simulink model "VSG1_RL"  (R2022a)
settings: Solver=FixedStepAuto  StartTime=0.5  StopTime=1  FixedStep=1e-6  RelTol=1e-3
values from neighbouring files (symbols this model uses):
  A5 = [0.002 0.002 0.002 0.002 0.002 0.002 0.002 0.002 0.002 0.002 0.002 0.002 ... (500 elements, 1x500)]    [Am.mat]
  Dmax = 50    [VSG_RL.m]
  Dmin = 20    [VSG_RL.m]
undefined symbols (not defined in the file or in its folder): sigbuilder_block
libraries: slpidlib x4, spsThreePhaseVIMeasurementLib x4, simulink x3, spsabctodq0Lib x3, spsThreePhaseSeriesRLCBranchLib x3, spsGroundLib x2, spsDCVoltageSourceLib x1, spsUniversalBridgeLib x1, powerlib_extras x1, rllib x1, spsThreePhaseSeriesRLCLoadLib x1, spsThreePhaseProgrammableVoltageSourceLib x1
settings Model: SimulationMode=accelerator  Creator=TC  LastModifiedBy=卢闯
settings SolverCC: ZeroCrossAlgorithm=Adaptive  AlgebraicLoopSolver=TrustRegion
settings DataIOCC: InitialState=xFinal  LoadInitialState=on  SaveOperatingPoint=on  SaveOutput=off  SignalLogging=off  DSMLogging=off  SaveTime=off
settings DebuggingCC: IgnoredZcDiagnostic=none  UnconnectedInputMsg=warning  UnconnectedOutputMsg=warning  UnconnectedLineMsg=warning  ArithmeticOperatorsInVariantConditions=warning
settings SFSimCC: CustomCodeUndefinedFunction=UseInterfaceOnly  SimTargetLang=C++  GPUAcceleration=on  SimDLTargetLibrary=cudnn
settings SimscapeCC: SimscapeLogLimitData=off

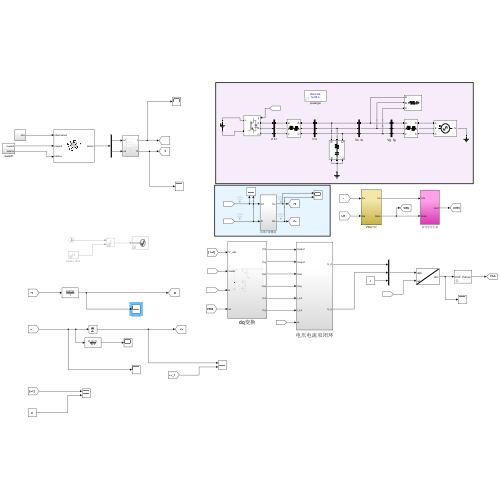
[thumbnail: Simulink's stored preview of the top-level diagram]
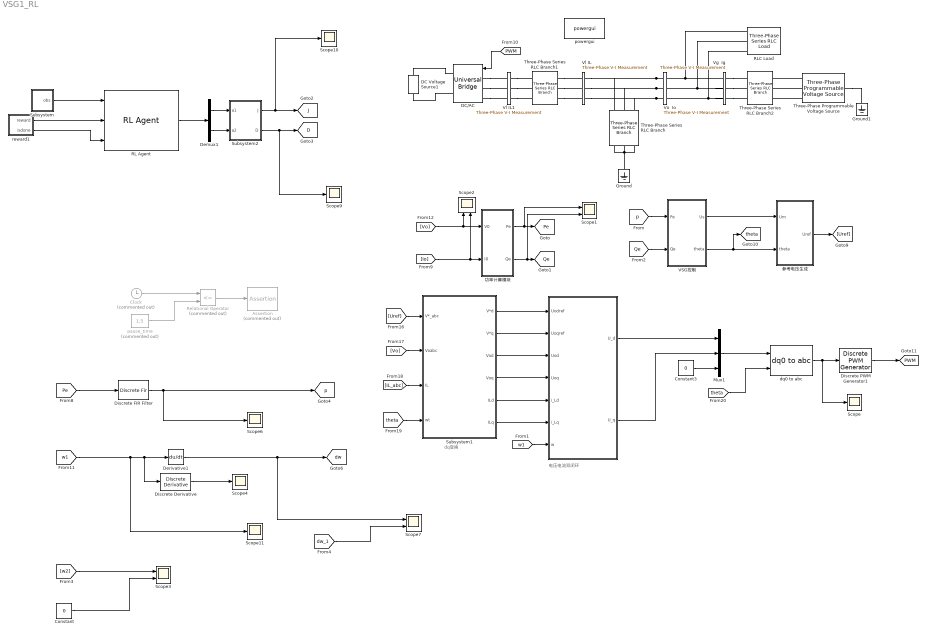
== system VSG1_RL ==
  note: 电压电流双闭环
  note: dq变换
  " " : Subsystem
  Assertion : Assertion  Commented=on  AssertionFailFcn=set_param(bdroot, 'SimulationCommand', 'pause')  StopWhenAssertionFail=off
  Clock : Clock  Commented=on
  Constant : Constant  Value=0
  Constant3 : Constant  Value=0
  DC Voltage Source1 : spsDCVoltageSourceLib/DC Voltage Source  Amplitude=750  Measurements=None
  DC/AC : spsUniversalBridgeLib/Universal Bridge  Arms=3  SnubberResistance=1e5  SnubberCapacitance=inf  Device=IGBT / Diodes  Ron=1e-3  Lon=0  ForwardVoltages="[  0  0  ]"  ForwardVoltage=0  GTOparameters=[ 10e-6 , 20e-6 ]  IGBTparameters=[ 1e-6 , 2e-6 ]  Measurements=None  Measurements_2=None  converterType=Rectifier
  Demux1 : Demux  Outputs=2
  Derivative1 : Derivative
  Discrete PWM Generator1 : powerlib_extras/Discrete  Control Blocks/Discrete PWM Generator  GeneratorMode="3-arm  bridge (6 pulses)"  Fc=10000  Ts=5e-6  Internal=off  mIndex=0.4  Freq=60  Phase=0
      settings: SourceProductBaseCode=PS
  Discrete Derivative : simulink/Discrete/Discrete Derivative  gainval=1.0  ICPrevScaledInput=0.0  OutMin=[]  OutMax=[]  OutDataType=fixdt(1, 16)  OutScaling=2^-10  DoSatur=off
  Discrete FIR Filter : DiscreteFir  Coefficients=A5
  Ground : spsGroundLib/Ground  LConnTagsString=a
  Ground1 : spsGroundLib/Ground  LConnTagsString=a
  Mux1 : Mux  Inputs=3
  RL Agent : rllib/RL Agent  Agent=agent  ExternalActionAsInput=off  ProvideLastAction=off  ProvideCumRwd=off  TreatAsDirectFeedthrough=on  UseStrictObservationDataTypes=off
  RLC Load : spsThreePhaseSeriesRLCLoadLib/Three-Phase Series RLC Load  LConnTagsString=A|B|C  Configuration=Y (grounded)  NominalVoltage=380  Vabc=[1e3 1e3 1e3]  Vabcp=[1e3 1e3 1e3]  NominalFrequency=50  UnbalancedPower=off  ActivePower=10e3  InductivePower=0  CapacitivePower=0  Pabc=[10e3 9e3 11e3]  QLabc=[100 90 110]  QCabc=[100 90 110]  Pabcp=[10e3 9e3 11e3]  QLabcp=[100 90 110]  QCabcp=[100 90 110]  Measurements=Branch voltages and currents  LoadType=constant Z
  Relational Operator : RelationalOperator  Commented=on  Operator=<=  OutDataTypeStr=boolean  RndMeth=Simplest  InputSameDT=off
  Scope{,4,6,9..11} (6 alike) : Scope
  Scope{1..3,7} (4 alike) : Scope  NumInputPorts=2
  Subsystem : Subsystem
  Subsystem1 : Subsystem
  Subsystem2 : Subsystem
  Three-Phase Programmable Voltage Source : spsThreePhaseProgrammableVoltageSourceLib/Three-Phase Programmable Voltage Source  PositiveSequence="[380  0 50]"  VariationEntity=None  VariationType=Table of time-amplitude pairs  VariationTypeAlt=Step  VariationStep=0.5  VariationRate=10  VariationMagnitude=0.3  VariationFrequency=2  VariationTiming=[1 2]  VariationPhaseA=off  Amplitudes=[1 0.8 1.2 1.0]  TimeValues=[0 0.1 0.15 0.2]  HarmonicGeneration=off  HarmonicA=[3 0.2 -25 0]  HarmonicB=[2 0.15 35 2]  Timing="[0.05  3]"  BusType=swing  Pref=0  Qref=0  Qmin=-inf  Qmax=inf
      link override Model/Signal generator/Stair Generator: t=[0.5,1,3,3.5]
  Three-Phase Series RLC Branch : spsThreePhaseSeriesRLCBranchLib/Three-Phase Series RLC Branch  LConnTagsString=A|B|C  RConnTagsString=A|B|C  BranchType=RC  Resistance=1  Inductance=1e-3  Capacitance=20e-6  Measurements=Branch voltages
  Three-Phase Series RLC Branch1 : spsThreePhaseSeriesRLCBranchLib/Three-Phase Series RLC Branch  LConnTagsString=A|B|C  RConnTagsString=A|B|C  BranchType=RL  Resistance=0.1  Inductance=3.2e-3  Capacitance=4.5e-3  Measurements=Branch voltages
  Three-Phase Series RLC Branch2 : spsThreePhaseSeriesRLCBranchLib/Three-Phase Series RLC Branch  LConnTagsString=A|B|C  RConnTagsString=A|B|C  BranchType=RL  Resistance=0.1  Inductance=3.0e-3  Capacitance=4.5e-3  Measurements=Branch voltages
  VSG控制 : Subsystem
  Vg  Ig : spsThreePhaseVIMeasurementLib/Three-Phase V-I Measurement  VoltageMeasurement=phase-to-ground  SetLabelV=on  LabelV=VGG  Vpu=off  VpuLL=off  CurrentMeasurement=yes  SetLabelI=on  LabelI=IGG  Ipu=off  Pbase=Pnom  Vbase=380  OutputType=Complex  PhasorSimulation=off  PSBequivalent=0
  Vl IL : spsThreePhaseVIMeasurementLib/Three-Phase V-I Measurement  VoltageMeasurement=phase-to-ground  SetLabelV=on  LabelV=VL_abc  Vpu=off  VpuLL=off  CurrentMeasurement=yes  SetLabelI=on  LabelI=IL_abc  Ipu=off  Pbase=100e6  Vbase=500e3  OutputType=Complex  PhasorSimulation=off  PSBequivalent=0
  Vl IL1 : spsThreePhaseVIMeasurementLib/Three-Phase V-I Measurement  VoltageMeasurement=phase-to-ground  SetLabelV=on  LabelV=VL  Vpu=off  VpuLL=off  CurrentMeasurement=yes  SetLabelI=on  LabelI=IL  Ipu=off  Pbase=100e6  Vbase=500e3  OutputType=Complex  PhasorSimulation=off  PSBequivalent=0
  Vo  Io : spsThreePhaseVIMeasurementLib/Three-Phase V-I Measurement  VoltageMeasurement=phase-to-ground  SetLabelV=on  LabelV=Vo  Vpu=off  VpuLL=off  CurrentMeasurement=yes  SetLabelI=on  LabelI=Io  Ipu=off  Pbase=Pnom  Vbase=380  OutputType=Complex  PhasorSimulation=off  PSBequivalent=0
  dq0 to abc : spsdq0toabcLib/dq0 to abc  Alignment=90 degrees behind phase A axis
  pause_time : Constant  Commented=on  Value=1.5
  powergui : spspowerguiLib/powergui  Priority=1  SimulationMode=Discrete  SampleTime=1e-6  frequency=60  Iterations=50  frequencyindice=0  Pbase=100e6  ErrMax=1e-4  UnitsV=kV  UnitsW=MW  buscounter=0  FunctionMessages=off  echomessages=off  EnableUseOfTLC=off  CurrentSourceSwitches=off  DisableSnubberDevices=off  DisableRonSwitches=off  DisableVfSwitches=off  DisplayEquations=off  AutomaticDiscreteSolvers=off  SolverType=Tustin/Backward Euler (TBE)  Interpol=off  ExternalGateDelay=off  methode=off  Ts=100  x0status=blocks  SPID=on  SwTol=0  HookPort=off  NonlinearTolerance=1e-4  nMaxIteration=100  ContinueOnMaxIteration=off  RestoreLinks=warning  ResistiveCurrentMeasurement=off  Frange=[0:2:500]  Ylog=off  Xlog=on  ShowGrid=off  save=off  variable=ZData  structure=0  ZoomFFT=off  StartTime=0.0  cycles=1  DisplayStyle=1  fundamental=60  FreqAxis=off  MaxFrequency=1000  frequencyindicesteady=1  RmsSteady=1  display=off
  reward1 : Subsystem
  功率计算模块 : Subsystem
  参考电压生成 : Subsystem
  tag scope: D=global, J=global, PWM=global, Pe=global, Qe=global, dw=global, p=global, theta=global
  wires:
  [PWM] -> DC/AC/1
  Mux1/1 -> dq0 to abc/1
  dq0 to abc/1 -> Scope/1, Discrete PWM Generator1/1
  " "/2(U_q) -> Mux1/2
  Discrete PWM Generator1/1 -> [PWM]
  参考电压生成/1(Uref) -> [Uref]
  [w1] -> " "/7(w)
  [IL_abc] -> Subsystem1/3(IL)
  [theta] -> Subsystem1/4(wt)
  Subsystem1/4(Voq) -> " "/4(Uoq)
  [Uref] -> Subsystem1/1(V*_abc)
  [theta] -> dq0 to abc/2
  [Io] -> 功率计算模块/2(I0), Scope2/2
  Constant3/1 -> Mux1/3
  " "/1(U_d) -> Mux1/1
  Subsystem1/1(V*d) -> " "/1(Uodref)
  [Vo] -> Subsystem1/2(Voabc)
  Subsystem1/2(V*q) -> " "/2(Uoqref)
  VSG控制/2(theta) -> 参考电压生成/2(theta), [theta]
  Subsystem1/5(ILd) -> " "/5(i_Ld)
  Subsystem1/3(Vod) -> " "/3(Uod)
  Subsystem1/6(ILq) -> " "/6(i_Lq)
  [Vo] -> 功率计算模块/1(V0), Scope2/1
  VSG控制/1(Us) -> 参考电压生成/1(Um)
  功率计算模块/1(Pe) -> Scope1/1, [Pe]
  功率计算模块/2(Qe) -> Scope1/2, [Qe]
  [p] -> VSG控制/1(Pe)
  [Qe] -> VSG控制/2(Qe)
  Clock/1 -> Relational Operator/1
  pause_time/1 -> Relational Operator/2
  Relational Operator/1 -> Assertion/1
  [w1] -> Discrete Derivative/1, Derivative1/1, Scope11/1
  [Pe] -> Discrete FIR Filter/1
  Discrete FIR Filter/1 -> [p], Scope6/1
  Subsystem2/2(D) -> Scope9/1, [D]
  Subsystem2/1(J) -> Scope10/1, [J]
  Demux1/1 -> Subsystem2/1(a1)
  Demux1/2 -> Subsystem2/2(a2)
  Subsystem/1(obs) -> RL Agent/1
  RL Agent/1 -> Demux1/1
  Derivative1/1 -> [dw], Scope7/1
  [w2] -> Scope3/1
  Constant/1 -> Scope3/2
  reward1/1(reward) -> RL Agent/2
  Discrete Derivative/1 -> Scope4/1
  [dw_1] -> Scope7/2
  reward1/2(isdone) -> RL Agent/3
  connections:
  Ground/LConn1 -- Three-Phase Series RLC Branch/RConn2 -- Three-Phase Series RLC Branch/RConn3 -- Three-Phase Series RLC Branch/RConn1
  Vo  Io/LConn2 -- Vl IL/RConn2 -- Three-Phase Series RLC Branch/LConn2
  Vo  Io/LConn3 -- Vl IL/RConn3 -- Three-Phase Series RLC Branch/LConn3
  Vo  Io/LConn1 -- Vl IL/RConn1 -- Three-Phase Series RLC Branch/LConn1
  Three-Phase Programmable Voltage Source/RConn3 -- Three-Phase Series RLC Branch2/LConn3
  Vg  Ig/LConn3 -- Vo  Io/RConn3 -- RLC Load/LConn3
  Three-Phase Programmable Voltage Source/RConn2 -- Three-Phase Series RLC Branch2/LConn2
  Three-Phase Series RLC Branch1/LConn2 -- Vl IL/LConn2
  Vg  Ig/LConn1 -- RLC Load/LConn1 -- Vo  Io/RConn1
  Three-Phase Programmable Voltage Source/RConn1 -- Three-Phase Series RLC Branch2/LConn1
  Three-Phase Programmable Voltage Source/LConn1 -- Ground1/LConn1
  Three-Phase Series RLC Branch1/LConn1 -- Vl IL/LConn1
  Vg  Ig/LConn2 -- RLC Load/LConn2 -- Vo  Io/RConn2
  Three-Phase Series RLC Branch1/LConn3 -- Vl IL/LConn3
  Vg  Ig/RConn1 -- Three-Phase Series RLC Branch2/RConn1
  Vg  Ig/RConn2 -- Three-Phase Series RLC Branch2/RConn2
  Vg  Ig/RConn3 -- Three-Phase Series RLC Branch2/RConn3
  DC Voltage Source1/RConn1 -- DC/AC/RConn1
  DC Voltage Source1/LConn1 -- DC/AC/RConn2
  DC/AC/LConn1 -- Vl IL1/LConn1
  Vl IL1/RConn1 -- Three-Phase Series RLC Branch1/RConn1
  DC/AC/LConn2 -- Vl IL1/LConn2
  Vl IL1/RConn2 -- Three-Phase Series RLC Branch1/RConn2
  DC/AC/LConn3 -- Vl IL1/LConn3
  Vl IL1/RConn3 -- Three-Phase Series RLC Branch1/RConn3

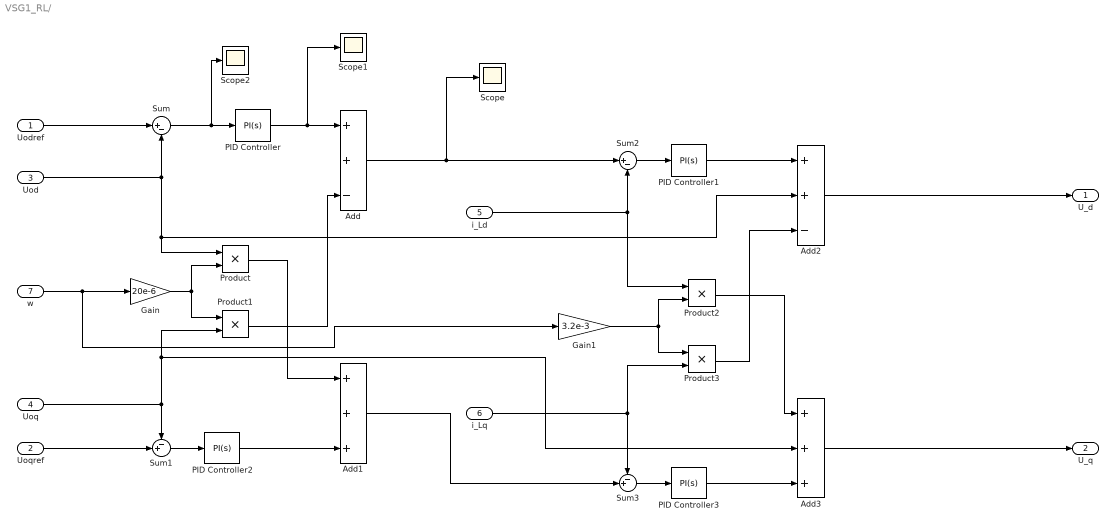
== system VSG1_RL/  ==
  Uodref : Inport
  Uoqref : Inport  Port=2
  Uod : Inport  Port=3
  Uoq : Inport  Port=4
  i_Ld : Inport  Port=5
  i_Lq : Inport  Port=6
  w : Inport  Port=7
  Add : Sum  Inputs=++-
  Add1 : Sum  Inputs=+++
  Add2 : Sum  Inputs=++-
  Add3 : Sum  Inputs=+++
  Gain : Gain  Gain=20e-6
  Gain1 : Gain  Gain=3.2e-3
  PID Controller : slpidlib/PID Controller  Controller=PI  Form=Parallel  TimeDomain=Continuous-time  UseExternalTs=off  SampleTime=1  IntegratorMethod=Forward Euler  FilterMethod=Forward Euler  ControllerParametersSource=internal  P=5  I=250  UseKiTs=off  D=0  N=100  UseFilter=on  TunerSelectOption=Transfer Function Based (PID Tuner App)  InitialConditionSource=internal  InitialConditionForIntegrator=0  InitialConditionForFilter=0  DifferentiatorICPrevScaledInput=0  ExternalReset=none  TrackingMode=off  Kt=1  LimitOutput=off  SatLimitsSource=internal  UpperSaturationLimit=inf  LowerSaturationLimit=-inf  LinearizeAsGain=off  AntiWindupMode=none  Kb=1  POutMin=[]  POutMax=[]  IOutMin=[]  IOutMax=[]  DOutMin=[]  DOutMax=[]  NOutMin=[]  NOutMax=[]  SumOutMin=[]  SumOutMax=[]  SaturationOutMin=[]  SaturationOutMax=[]  PParamMin=[]  PParamMax=[]  IParamMin=[]  IParamMax=[]  DParamMin=[]  DParamMax=[]  NParamMin=[]  NParamMax=[]  KbParamMin=[]  KbParamMax=[]  KtParamMin=[]  KtParamMax=[]  KbOutMin=[]  KbOutMax=[]  KtOutMin=[]  KtOutMax=[]  IntegratorOutMin=[]  IntegratorOutMax=[]  FilterOutMin=[]  FilterOutMax=[]  SumI1OutMin=[]  SumI1OutMax=[]  SumI2OutMin=[]  SumI2OutMax=[]  SumI3OutMin=[]  SumI3OutMax=[]  SumI4OutMin=[]  SumI4OutMax=[]  SumDOutMin=[]  SumDOutMax=[]  DifferentiatorOutMin=[]  DifferentiatorOutMax=[]  FilterDiffOutCoefMin=[]  FilterDiffOutCoefMax=[]  ReciprocalOutMin=[]  ReciprocalOutMax=[]  SumDenOutMin=[]  SumDenOutMax=[]  SumNumOutMin=[]  SumNumOutMax=[]  DivideOutMin=[]  DivideOutMax=[]  UdiffTsProdOutMin=[]  UdiffTsProdOutMax=[]  NTsProdOutMin=[]  NTsProdOutMax=[]  UintegralTsProdOutMin=[]  UintegralTsProdOutMax=[]  UngainTsProdOutMin=[]  UngainTsProdOutMax=[]  ClampingZeroOutDataTypeStr=Inherit: Inherit via back propagation  ClampingZeroOutMin=[]  ClampingZeroOutMax=[]  FilterDenConstantOutDataTypeStr=Inherit: Inherit via back propagation  FilterDenConstantOutMin=[]  FilterDenConstantOutMax=[]  PCopyOutDataTypeStr=Inherit: Inherit via back propagation  PCopyOutMin=[]  PCopyOutMax=[]  NCopyOutDataTypeStr=Inherit: Inherit via back propagation  NCopyOutMin=[]  NCopyOutMax=[]  IntegratorContinuousStateAttributes=''  IntegratorStateMustResolveToSignalObject=off  IntegratorRTWStateStorageClass=Auto  FilterContinuousStateAttributes=''  FilterStateMustResolveToSignalObject=off  FilterRTWStateStorageClass=Auto  ParallelPVariant=InternalParameters  IdealPVariant=Disabled  IVariant=InternalParameters  DVariant=Disabled  IntegratorVariant=Continuous  SatVariant=Disabled  AWVariant=Passthrough  PCopyVariant=Disabled  TRVariant=Disabled  FdbkBlocksVariant=Forward  IdealPFdbkVariant=Disabled  SatFdbkVariant=Disabled  DerivativeFilterVariant=Disabled  NVariant=Disabled  NCopyVariant=Disabled_SignalSpec  FilterICVariant=Disabled  IntegratorICVariant=InternalICs  ExternalResetVariant=Disabled  TRSumVariant=Passthrough  SumFdbkVariant=Disabled  SumVariant=Sum_PI  TsampFilterVariant=InternalTs  TsampNgainVariant=Passthrough  TsampIntegralVariant=Passthrough  ExternalSaturationOutDataTypeStr=Inherit: Same as second input  aMode=0
  PID Controller1 : slpidlib/PID Controller  Controller=PI  Form=Parallel  TimeDomain=Continuous-time  UseExternalTs=off  SampleTime=1  IntegratorMethod=Forward Euler  FilterMethod=Forward Euler  ControllerParametersSource=internal  P=20  I=200  UseKiTs=off  D=0  N=100  UseFilter=on  TunerSelectOption=Transfer Function Based (PID Tuner App)  InitialConditionSource=internal  InitialConditionForIntegrator=0  InitialConditionForFilter=0  DifferentiatorICPrevScaledInput=0  ExternalReset=none  TrackingMode=off  Kt=1  LimitOutput=off  SatLimitsSource=internal  UpperSaturationLimit=inf  LowerSaturationLimit=-inf  LinearizeAsGain=off  AntiWindupMode=none  Kb=1  POutMin=[]  POutMax=[]  IOutMin=[]  IOutMax=[]  DOutMin=[]  DOutMax=[]  NOutMin=[]  NOutMax=[]  SumOutMin=[]  SumOutMax=[]  SaturationOutMin=[]  SaturationOutMax=[]  PParamMin=[]  PParamMax=[]  IParamMin=[]  IParamMax=[]  DParamMin=[]  DParamMax=[]  NParamMin=[]  NParamMax=[]  KbParamMin=[]  KbParamMax=[]  KtParamMin=[]  KtParamMax=[]  KbOutMin=[]  KbOutMax=[]  KtOutMin=[]  KtOutMax=[]  IntegratorOutMin=[]  IntegratorOutMax=[]  FilterOutMin=[]  FilterOutMax=[]  SumI1OutMin=[]  SumI1OutMax=[]  SumI2OutMin=[]  SumI2OutMax=[]  SumI3OutMin=[]  SumI3OutMax=[]  SumI4OutMin=[]  SumI4OutMax=[]  SumDOutMin=[]  SumDOutMax=[]  DifferentiatorOutMin=[]  DifferentiatorOutMax=[]  FilterDiffOutCoefMin=[]  FilterDiffOutCoefMax=[]  ReciprocalOutMin=[]  ReciprocalOutMax=[]  SumDenOutMin=[]  SumDenOutMax=[]  SumNumOutMin=[]  SumNumOutMax=[]  DivideOutMin=[]  DivideOutMax=[]  UdiffTsProdOutMin=[]  UdiffTsProdOutMax=[]  NTsProdOutMin=[]  NTsProdOutMax=[]  UintegralTsProdOutMin=[]  UintegralTsProdOutMax=[]  UngainTsProdOutMin=[]  UngainTsProdOutMax=[]  ClampingZeroOutDataTypeStr=Inherit: Inherit via back propagation  ClampingZeroOutMin=[]  ClampingZeroOutMax=[]  FilterDenConstantOutDataTypeStr=Inherit: Inherit via back propagation  FilterDenConstantOutMin=[]  FilterDenConstantOutMax=[]  PCopyOutDataTypeStr=Inherit: Inherit via back propagation  PCopyOutMin=[]  PCopyOutMax=[]  NCopyOutDataTypeStr=Inherit: Inherit via back propagation  NCopyOutMin=[]  NCopyOutMax=[]  IntegratorContinuousStateAttributes=''  IntegratorStateMustResolveToSignalObject=off  IntegratorRTWStateStorageClass=Auto  FilterContinuousStateAttributes=''  FilterStateMustResolveToSignalObject=off  FilterRTWStateStorageClass=Auto  ParallelPVariant=InternalParameters  IdealPVariant=Disabled  IVariant=InternalParameters  DVariant=Disabled  IntegratorVariant=Continuous  SatVariant=Disabled  AWVariant=Passthrough  PCopyVariant=Disabled  TRVariant=Disabled  FdbkBlocksVariant=Forward  IdealPFdbkVariant=Disabled  SatFdbkVariant=Disabled  DerivativeFilterVariant=Disabled  NVariant=Disabled  NCopyVariant=Disabled_SignalSpec  FilterICVariant=Disabled  IntegratorICVariant=InternalICs  ExternalResetVariant=Disabled  TRSumVariant=Passthrough  SumFdbkVariant=Disabled  SumVariant=Sum_PI  TsampFilterVariant=InternalTs  TsampNgainVariant=Passthrough  TsampIntegralVariant=Passthrough  ExternalSaturationOutDataTypeStr=Inherit: Same as second input  aMode=0
  PID Controller2 : slpidlib/PID Controller  Controller=PI  Form=Parallel  TimeDomain=Continuous-time  UseExternalTs=off  SampleTime=1  IntegratorMethod=Forward Euler  FilterMethod=Forward Euler  ControllerParametersSource=internal  P=5  I=250  UseKiTs=off  D=0  N=100  UseFilter=on  TunerSelectOption=Transfer Function Based (PID Tuner App)  InitialConditionSource=internal  InitialConditionForIntegrator=0  InitialConditionForFilter=0  DifferentiatorICPrevScaledInput=0  ExternalReset=none  TrackingMode=off  Kt=1  LimitOutput=off  SatLimitsSource=internal  UpperSaturationLimit=inf  LowerSaturationLimit=-inf  LinearizeAsGain=off  AntiWindupMode=none  Kb=1  POutMin=[]  POutMax=[]  IOutMin=[]  IOutMax=[]  DOutMin=[]  DOutMax=[]  NOutMin=[]  NOutMax=[]  SumOutMin=[]  SumOutMax=[]  SaturationOutMin=[]  SaturationOutMax=[]  PParamMin=[]  PParamMax=[]  IParamMin=[]  IParamMax=[]  DParamMin=[]  DParamMax=[]  NParamMin=[]  NParamMax=[]  KbParamMin=[]  KbParamMax=[]  KtParamMin=[]  KtParamMax=[]  KbOutMin=[]  KbOutMax=[]  KtOutMin=[]  KtOutMax=[]  IntegratorOutMin=[]  IntegratorOutMax=[]  FilterOutMin=[]  FilterOutMax=[]  SumI1OutMin=[]  SumI1OutMax=[]  SumI2OutMin=[]  SumI2OutMax=[]  SumI3OutMin=[]  SumI3OutMax=[]  SumI4OutMin=[]  SumI4OutMax=[]  SumDOutMin=[]  SumDOutMax=[]  DifferentiatorOutMin=[]  DifferentiatorOutMax=[]  FilterDiffOutCoefMin=[]  FilterDiffOutCoefMax=[]  ReciprocalOutMin=[]  ReciprocalOutMax=[]  SumDenOutMin=[]  SumDenOutMax=[]  SumNumOutMin=[]  SumNumOutMax=[]  DivideOutMin=[]  DivideOutMax=[]  UdiffTsProdOutMin=[]  UdiffTsProdOutMax=[]  NTsProdOutMin=[]  NTsProdOutMax=[]  UintegralTsProdOutMin=[]  UintegralTsProdOutMax=[]  UngainTsProdOutMin=[]  UngainTsProdOutMax=[]  ClampingZeroOutDataTypeStr=Inherit: Inherit via back propagation  ClampingZeroOutMin=[]  ClampingZeroOutMax=[]  FilterDenConstantOutDataTypeStr=Inherit: Inherit via back propagation  FilterDenConstantOutMin=[]  FilterDenConstantOutMax=[]  PCopyOutDataTypeStr=Inherit: Inherit via back propagation  PCopyOutMin=[]  PCopyOutMax=[]  NCopyOutDataTypeStr=Inherit: Inherit via back propagation  NCopyOutMin=[]  NCopyOutMax=[]  IntegratorContinuousStateAttributes=''  IntegratorStateMustResolveToSignalObject=off  IntegratorRTWStateStorageClass=Auto  FilterContinuousStateAttributes=''  FilterStateMustResolveToSignalObject=off  FilterRTWStateStorageClass=Auto  ParallelPVariant=InternalParameters  IdealPVariant=Disabled  IVariant=InternalParameters  DVariant=Disabled  IntegratorVariant=Continuous  SatVariant=Disabled  AWVariant=Passthrough  PCopyVariant=Disabled  TRVariant=Disabled  FdbkBlocksVariant=Forward  IdealPFdbkVariant=Disabled  SatFdbkVariant=Disabled  DerivativeFilterVariant=Disabled  NVariant=Disabled  NCopyVariant=Disabled_SignalSpec  FilterICVariant=Disabled  IntegratorICVariant=InternalICs  ExternalResetVariant=Disabled  TRSumVariant=Passthrough  SumFdbkVariant=Disabled  SumVariant=Sum_PI  TsampFilterVariant=InternalTs  TsampNgainVariant=Passthrough  TsampIntegralVariant=Passthrough  ExternalSaturationOutDataTypeStr=Inherit: Same as second input  aMode=0
  PID Controller3 : slpidlib/PID Controller  Controller=PI  Form=Parallel  TimeDomain=Continuous-time  UseExternalTs=off  SampleTime=1  IntegratorMethod=Forward Euler  FilterMethod=Forward Euler  ControllerParametersSource=internal  P=20  I=200  UseKiTs=off  D=0  N=100  UseFilter=on  TunerSelectOption=Transfer Function Based (PID Tuner App)  InitialConditionSource=internal  InitialConditionForIntegrator=0  InitialConditionForFilter=0  DifferentiatorICPrevScaledInput=0  ExternalReset=none  TrackingMode=off  Kt=1  LimitOutput=off  SatLimitsSource=internal  UpperSaturationLimit=inf  LowerSaturationLimit=-inf  LinearizeAsGain=off  AntiWindupMode=none  Kb=1  POutMin=[]  POutMax=[]  IOutMin=[]  IOutMax=[]  DOutMin=[]  DOutMax=[]  NOutMin=[]  NOutMax=[]  SumOutMin=[]  SumOutMax=[]  SaturationOutMin=[]  SaturationOutMax=[]  PParamMin=[]  PParamMax=[]  IParamMin=[]  IParamMax=[]  DParamMin=[]  DParamMax=[]  NParamMin=[]  NParamMax=[]  KbParamMin=[]  KbParamMax=[]  KtParamMin=[]  KtParamMax=[]  KbOutMin=[]  KbOutMax=[]  KtOutMin=[]  KtOutMax=[]  IntegratorOutMin=[]  IntegratorOutMax=[]  FilterOutMin=[]  FilterOutMax=[]  SumI1OutMin=[]  SumI1OutMax=[]  SumI2OutMin=[]  SumI2OutMax=[]  SumI3OutMin=[]  SumI3OutMax=[]  SumI4OutMin=[]  SumI4OutMax=[]  SumDOutMin=[]  SumDOutMax=[]  DifferentiatorOutMin=[]  DifferentiatorOutMax=[]  FilterDiffOutCoefMin=[]  FilterDiffOutCoefMax=[]  ReciprocalOutMin=[]  ReciprocalOutMax=[]  SumDenOutMin=[]  SumDenOutMax=[]  SumNumOutMin=[]  SumNumOutMax=[]  DivideOutMin=[]  DivideOutMax=[]  UdiffTsProdOutMin=[]  UdiffTsProdOutMax=[]  NTsProdOutMin=[]  NTsProdOutMax=[]  UintegralTsProdOutMin=[]  UintegralTsProdOutMax=[]  UngainTsProdOutMin=[]  UngainTsProdOutMax=[]  ClampingZeroOutDataTypeStr=Inherit: Inherit via back propagation  ClampingZeroOutMin=[]  ClampingZeroOutMax=[]  FilterDenConstantOutDataTypeStr=Inherit: Inherit via back propagation  FilterDenConstantOutMin=[]  FilterDenConstantOutMax=[]  PCopyOutDataTypeStr=Inherit: Inherit via back propagation  PCopyOutMin=[]  PCopyOutMax=[]  NCopyOutDataTypeStr=Inherit: Inherit via back propagation  NCopyOutMin=[]  NCopyOutMax=[]  IntegratorContinuousStateAttributes=''  IntegratorStateMustResolveToSignalObject=off  IntegratorRTWStateStorageClass=Auto  FilterContinuousStateAttributes=''  FilterStateMustResolveToSignalObject=off  FilterRTWStateStorageClass=Auto  ParallelPVariant=InternalParameters  IdealPVariant=Disabled  IVariant=InternalParameters  DVariant=Disabled  IntegratorVariant=Continuous  SatVariant=Disabled  AWVariant=Passthrough  PCopyVariant=Disabled  TRVariant=Disabled  FdbkBlocksVariant=Forward  IdealPFdbkVariant=Disabled  SatFdbkVariant=Disabled  DerivativeFilterVariant=Disabled  NVariant=Disabled  NCopyVariant=Disabled_SignalSpec  FilterICVariant=Disabled  IntegratorICVariant=InternalICs  ExternalResetVariant=Disabled  TRSumVariant=Passthrough  SumFdbkVariant=Disabled  SumVariant=Sum_PI  TsampFilterVariant=InternalTs  TsampNgainVariant=Passthrough  TsampIntegralVariant=Passthrough  ExternalSaturationOutDataTypeStr=Inherit: Same as second input  aMode=0
  Product{,1..3} (4 alike) : Product  RndMeth=Zero
  Scope : Scope
  Scope1 : Scope
  Scope2 : Scope
  Sum : Sum  Inputs=|+-
  Sum1 : Sum  Inputs=-+|
  Sum2 : Sum  Inputs=|+-
  Sum3 : Sum  Inputs=-+|
  U_d : Outport  VectorParamsAs1DForOutWhenUnconnected=off
  U_q : Outport  Port=2  VectorParamsAs1DForOutWhenUnconnected=off
  wires:
  Uod/1 -> Sum/2, Add2/2, Product/1
  Add/1 -> Scope/1, Sum2/1
  i_Lq/1 -> Sum3/1, Product3/2
  i_Ld/1 -> Sum2/2, Product2/1
  Sum2/1 -> PID Controller1/1
  PID Controller1/1 -> Add2/1
  Add1/1 -> Sum3/2
  Product2/1 -> Add3/1
  Product3/1 -> Add2/3
  Gain/1 -> Product1/1, Product/2
  Gain1/1 -> Product3/1, Product2/2
  Uoq/1 -> Sum1/1, Product1/2, Add3/2
  PID Controller3/1 -> Add3/3
  Sum3/1 -> PID Controller3/1
  Product1/1 -> Add/3
  Product/1 -> Add1/1
  PID Controller2/1 -> Add1/3
  Sum1/1 -> PID Controller2/1
  PID Controller/1 -> Scope1/1, Add/1
  w/1 -> Gain1/1, Gain/1
  Uoqref/1 -> Sum1/2
  Uodref/1 -> Sum/1
  Sum/1 -> Scope2/1, PID Controller/1
  Add2/1 -> U_d/1
  Add3/1 -> U_q/1

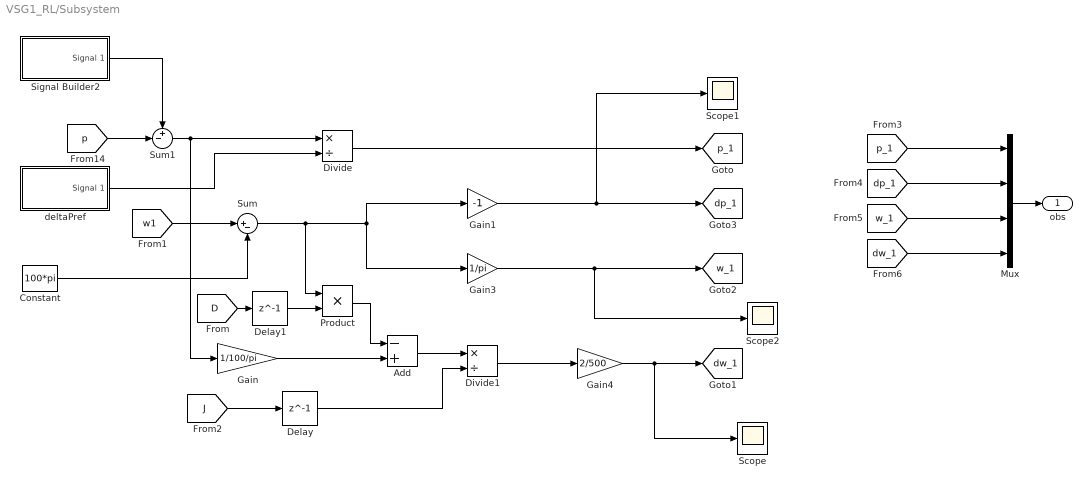
== system VSG1_RL/Subsystem ==
  Add : Sum  Inputs=-+
  Constant : Constant  Value=100*pi
  Delay : Delay  DelayLength=1  InitialCondition=0.02  SampleTime=0.0005
  Delay1 : Delay  DelayLength=1  SampleTime=0.0005
  Divide : Product  Inputs=*/
  Divide1 : Product  Inputs=*/
  Gain : Gain  Gain=1/100/pi
  Gain1 : Gain  Gain=-1
  Gain3 : Gain  Gain=1/pi
  Gain4 : Gain  Gain=2/500
  Mux : Mux
  Product : Product
  Scope : Scope
  Scope1 : Scope
  Scope2 : Scope
  Signal Builder2 : Subsystem  Tag=STV Subsys  LoadFcn=sigbuilder_block('load');  StartFcn=sigbuilder_block('start');  StopFcn=sigbuilder_block('stop');  ClipboardFcn=sigbuilder_block('clipboard');  mask(Sigbuilder block){tuvar=[0:10]}
      mask help: Simulink:masks:SigbuilderBlock_MD
      mask init:
      | if ~strcmp(get_param(bdroot(gcbh),'SimulationStatus'),'stopped') tuvar = sigbuilder_block('maskInit'); end
      settings: CopyFcn=sigbuilder_block('copy');  DeleteFcn=sigbuilder_block('delete');  ModelCloseFcn=sigbuilder_block('modelClose');  PreSaveFcn=sigbuilder_block('preSave');  PauseFcn=sigbuilder_block('pause');  ContinueFcn=sigbuilder_block('continue');  NameChangeFcn=sigbuilder_block('namechange');  OpenFcn=sigbuilder_block('open',[63 119.25 1012.5 505.5 ]);  CloseFcn=sigbuilder_block('close');
      mask Display: plot(0, 0, 100, 100,[2, 2, 32, 32, 2], [68, 8, 8, 68, 68],[32, 2], [38, 38], [32, 19, 2],[53, 60, 44], [32, 17, 17, 2],[16, 16, 31, 31]);txt = getActiveGroup(gcbh);text(2, 100, txt,'verticalAlignment', 'top');
  Sum : Sum  Inputs=|+-
  Sum1 : Sum  Inputs=+-|
  deltaPref : Subsystem  Tag=STV Subsys  LoadFcn=sigbuilder_block('load');  StartFcn=sigbuilder_block('start');  StopFcn=sigbuilder_block('stop');  ClipboardFcn=sigbuilder_block('clipboard');  mask(Sigbuilder block){tuvar=[0:10]}
      mask help: Simulink:masks:SigbuilderBlock_MD
      mask init:
      | if ~strcmp(get_param(bdroot(gcbh),'SimulationStatus'),'stopped') tuvar = sigbuilder_block('maskInit'); end
      settings: CopyFcn=sigbuilder_block('copy');  DeleteFcn=sigbuilder_block('delete');  ModelCloseFcn=sigbuilder_block('modelClose');  PreSaveFcn=sigbuilder_block('preSave');  PauseFcn=sigbuilder_block('pause');  ContinueFcn=sigbuilder_block('continue');  NameChangeFcn=sigbuilder_block('namechange');  OpenFcn=sigbuilder_block('open',[63 119.25 1012.5 505.5 ]);  CloseFcn=sigbuilder_block('close');
      mask Display: plot(0, 0, 100, 100,[2, 2, 32, 32, 2], [68, 8, 8, 68, 68],[32, 2], [38, 38], [32, 19, 2],[53, 60, 44], [32, 17, 17, 2],[16, 16, 31, 31]);txt = getActiveGroup(gcbh);text(2, 100, txt,'verticalAlignment', 'top');
  obs : Outport
  tag scope: dp_1=global, dw_1=global, p_1=global, w_1=global
  wires:
  Signal Builder2/1(Signal 1) -> Sum1/1
  [p] -> Sum1/2
  Mux/1 -> obs/1
  [w1] -> Sum/1
  Sum/1 -> Product/1, Gain1/1, Gain3/1
  Constant/1 -> Sum/2
  Gain3/1 -> Scope2/1, [w_1]
  Sum1/1 -> Gain/1, Divide/1
  deltaPref/1(Signal 1) -> Divide/2
  Divide/1 -> [p_1]
  [D] -> Delay1/1
  Gain/1 -> Add/2
  Product/1 -> Add/1
  Add/1 -> Divide1/1
  [J] -> Delay/1
  Gain1/1 -> Scope1/1, [dp_1]
  Divide1/1 -> Gain4/1
  [p_1] -> Mux/1
  [dp_1] -> Mux/2
  [w_1] -> Mux/3
  [dw_1] -> Mux/4
  Delay/1 -> Divide1/2
  Delay1/1 -> Product/2
  Gain4/1 -> Scope/1, [dw_1]

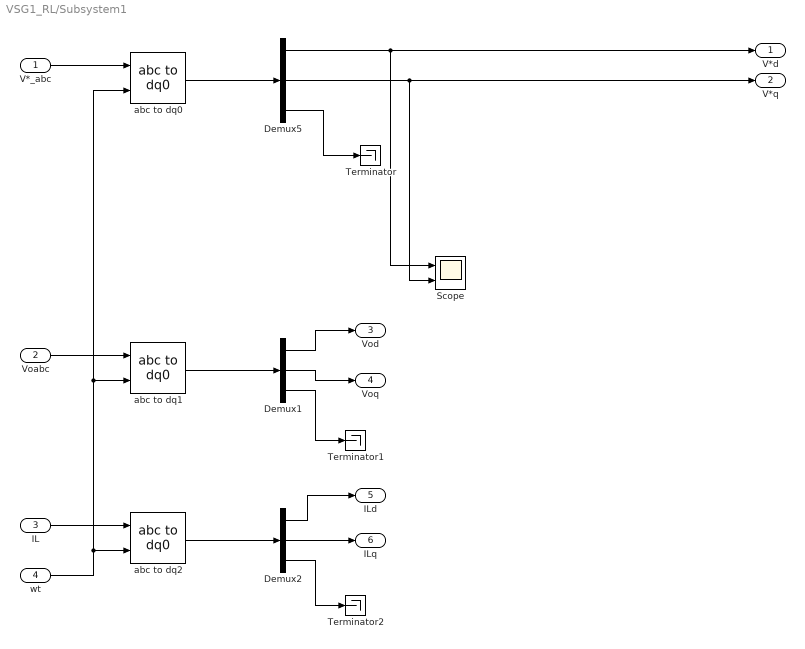
== system VSG1_RL/Subsystem1 ==
  V*_abc : Inport
  Voabc : Inport  Port=2
  IL : Inport  Port=3
  wt : Inport  Port=4
  Demux1 : Demux  Outputs=3
  Demux2 : Demux  Outputs=3
  Demux5 : Demux  Outputs=3
  Scope : Scope  NumInputPorts=2
  Terminator : Terminator
  Terminator1 : Terminator
  Terminator2 : Terminator
  abc to dq0 : spsabctodq0Lib/abc to dq0  Alignment=90 degrees behind phase A axis
  abc to dq1 : spsabctodq0Lib/abc to dq0  Alignment=90 degrees behind phase A axis
  abc to dq2 : spsabctodq0Lib/abc to dq0  Alignment=90 degrees behind phase A axis
  V*d : Outport  VectorParamsAs1DForOutWhenUnconnected=off
  V*q : Outport  Port=2  VectorParamsAs1DForOutWhenUnconnected=off
  Vod : Outport  Port=3  VectorParamsAs1DForOutWhenUnconnected=off
  Voq : Outport  Port=4  VectorParamsAs1DForOutWhenUnconnected=off
  ILd : Outport  Port=5  VectorParamsAs1DForOutWhenUnconnected=off
  ILq : Outport  Port=6  VectorParamsAs1DForOutWhenUnconnected=off
  wires:
  Demux5/2 -> V*q/1, Scope/2
  Demux5/1 -> V*d/1, Scope/1
  IL/1 -> abc to dq2/1
  Demux2/2 -> ILq/1
  Demux1/2 -> Voq/1
  Demux1/1 -> Vod/1
  Demux2/3 -> Terminator2/1
  Demux5/3 -> Terminator/1
  V*_abc/1 -> abc to dq0/1
  wt/1 -> abc to dq0/2, abc to dq1/2, abc to dq2/2
  Voabc/1 -> abc to dq1/1
  abc to dq1/1 -> Demux1/1
  abc to dq2/1 -> Demux2/1
  Demux1/3 -> Terminator1/1
  abc to dq0/1 -> Demux5/1
  Demux2/1 -> ILd/1

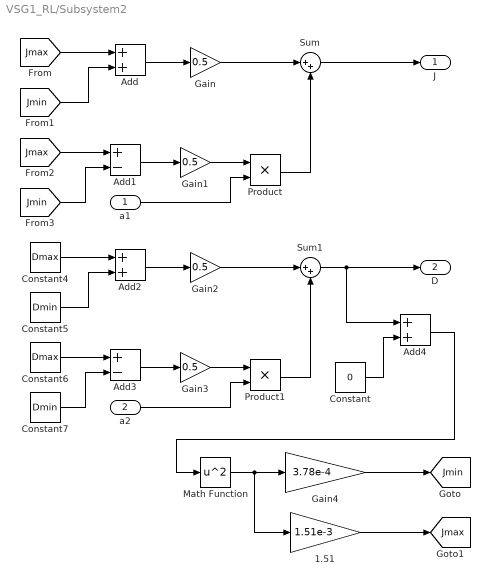
== system VSG1_RL/Subsystem2 ==
  a1 : Inport
  a2 : Inport  Port=2
  1.51 : Gain  Gain=1.51e-3
  Add : Sum
  Add1 : Sum  Inputs=+-
  Add2 : Sum
  Add3 : Sum  Inputs=+-
  Add4 : Sum
  Constant : Constant  Value=0
  Constant4 : Constant  Value=Dmax
  Constant5 : Constant  Value=Dmin
  Constant6 : Constant  Value=Dmax
  Constant7 : Constant  Value=Dmin
  Gain{,1..3} (4 alike) : Gain  Gain=0.5
  Gain4 : Gain  Gain=3.78e-4
  Math Function : Math  Operator=square
  Product : Product
  Product1 : Product
  Sum : Sum  Inputs=|++
  Sum1 : Sum  Inputs=|++
  J : Outport
  D : Outport  Port=2
  tag scope: Jmax=global, Jmin=global
  wires:
  [Jmax] -> Add/1
  [Jmin] -> Add/2
  Add/1 -> Gain/1
  Gain/1 -> Sum/1
  Add1/1 -> Gain1/1
  [Jmax] -> Add1/1
  [Jmin] -> Add1/2
  Gain1/1 -> Product/1
  a1/1 -> Product/2
  Product/1 -> Sum/2
  Product1/1 -> Sum1/2
  a2/1 -> Product1/2
  Gain3/1 -> Product1/1
  Constant7/1 -> Add3/2
  Constant6/1 -> Add3/1
  Add3/1 -> Gain3/1
  Gain2/1 -> Sum1/1
  Add2/1 -> Gain2/1
  Constant5/1 -> Add2/2
  Constant4/1 -> Add2/1
  Sum/1 -> J/1
  Sum1/1 -> Add4/1, D/1
  Math Function/1 -> 1.51/1, Gain4/1
  Gain4/1 -> [Jmin]
  1.51/1 -> [Jmax]
  Constant/1 -> Add4/2
  Add4/1 -> Math Function/1

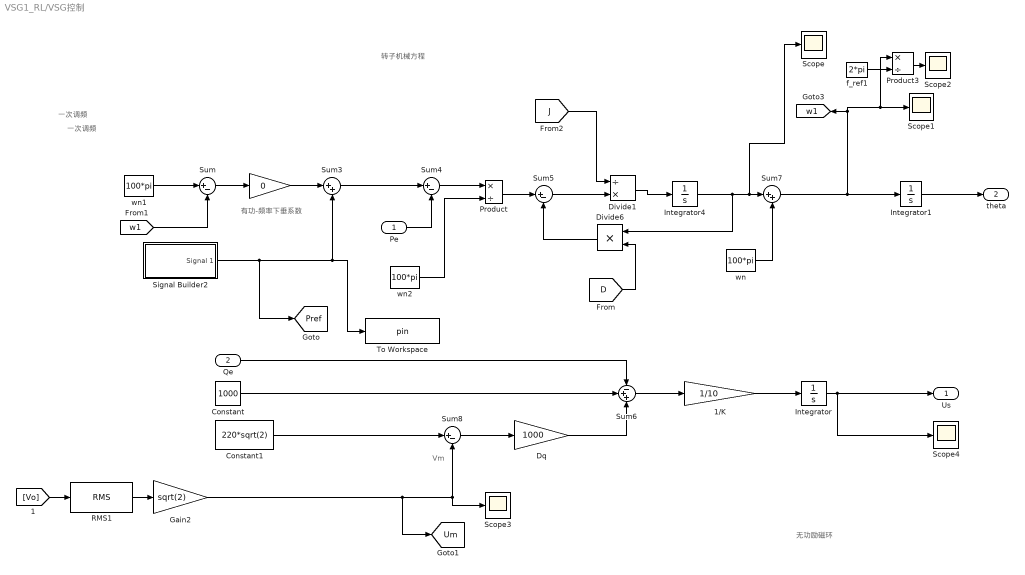
== system VSG1_RL/VSG控制 ==
  note: 无功励磁环
  note: 一次调频
  note: 转子机械方程
  note: 一次调频
  note: 有功-频率下垂系数
  note: Vm
  Pe : Inport
  Qe : Inport  Port=2
  " " : Gain  Gain=0
  1/K : Gain  Gain=1/10
  Constant : Constant  Value=1000
  Constant1 : Constant  Value=220*sqrt(2)
  Divide1 : Product  Inputs=/*
  Divide6 : Product  Inputs=**
  Dq : Gain  Gain=1000
  Gain2 : Gain  Gain=sqrt(2)
  Integrator : Integrator  InitialCondition=0.99
  Integrator1 : Integrator
  Integrator4 : Integrator
  Product : Product  Inputs=*/
  Product3 : Product  Inputs=*/
  RMS1 : dspstat3/RMS  run=off  directionMode=Each column  dimension=1  InputProcessing=Columns as channels (frame based)  reset_popup=None
  Scope{,1..4} (5 alike) : Scope
  Signal Builder2 : Subsystem  Tag=STV Subsys  LoadFcn=sigbuilder_block('load');  StartFcn=sigbuilder_block('start');  StopFcn=sigbuilder_block('stop');  ClipboardFcn=sigbuilder_block('clipboard');  mask(Sigbuilder block){tuvar=[0:10]}
      mask help: Simulink:masks:SigbuilderBlock_MD
      mask init:
      | if ~strcmp(get_param(bdroot(gcbh),'SimulationStatus'),'stopped') tuvar = sigbuilder_block('maskInit'); end
      settings: CopyFcn=sigbuilder_block('copy');  DeleteFcn=sigbuilder_block('delete');  ModelCloseFcn=sigbuilder_block('modelClose');  PreSaveFcn=sigbuilder_block('preSave');  PauseFcn=sigbuilder_block('pause');  ContinueFcn=sigbuilder_block('continue');  NameChangeFcn=sigbuilder_block('namechange');  OpenFcn=sigbuilder_block('open',[63 119.25 1012.5 505.5 ]);  CloseFcn=sigbuilder_block('close');
      mask Display: plot(0, 0, 100, 100,[2, 2, 32, 32, 2], [68, 8, 8, 68, 68],[32, 2], [38, 38], [32, 19, 2],[53, 60, 44], [32, 17, 17, 2],[16, 16, 31, 31]);txt = getActiveGroup(gcbh);text(2, 100, txt,'verticalAlignment', 'top');
  Sum{,4..5,8} (4 alike) : Sum  Inputs=|+-
  Sum3 : Sum  Inputs=|++
  Sum6 : Sum  Inputs=-++
  Sum7 : Sum  Inputs=|++
  To Workspace : ToWorkspace  VariableName=pin  SampleTime=1e-6
  f_ref1 : Constant  Value=2*pi
  wn : Constant  Value=100*pi
  wn1 : Constant  Value=100*pi
  wn2 : Constant  Value=100*pi
  Us : Outport  VectorParamsAs1DForOutWhenUnconnected=off
  theta : Outport  Port=2  VectorParamsAs1DForOutWhenUnconnected=off
  tag scope: Pref=global, Um=global, w1=global
  wires:
  Product/1 -> Sum5/1
  " "/1 -> Sum3/1
  Sum/1 -> " "/1
  Constant/1 -> Sum6/2
  wn/1 -> Sum7/2
  RMS1/1 -> Gain2/1
  Qe/1 -> Sum6/1
  1/K/1 -> Integrator/1
  wn2/1 -> Product/2
  Divide6/1 -> Sum5/2
  Sum4/1 -> Product/1
  wn1/1 -> Sum/1
  Constant1/1 -> Sum8/1
  Sum8/1 -> Dq/1
  Sum6/1 -> 1/K/1
  Divide1/1 -> Integrator4/1
  [w1] -> Sum/2
  Dq/1 -> Sum6/3
  Pe/1 -> Sum4/2
  Sum3/1 -> Sum4/1
  Integrator/1 -> Us/1, Scope4/1
  [Vo] -> RMS1/1
  Sum5/1 -> Divide1/2
  Integrator1/1 -> theta/1
  f_ref1/1 -> Product3/2
  Product3/1 -> Scope2/1
  Integrator4/1 -> Divide6/1, Scope/1, Sum7/1
  Sum7/1 -> Product3/1, Scope1/1, [w1], Integrator1/1
  Signal Builder2/1(Signal 1) -> [Pref], To Workspace/1, Sum3/2
  [J] -> Divide1/1
  [D] -> Divide6/2
  Gain2/1 -> [Um], Sum8/2, Scope3/1

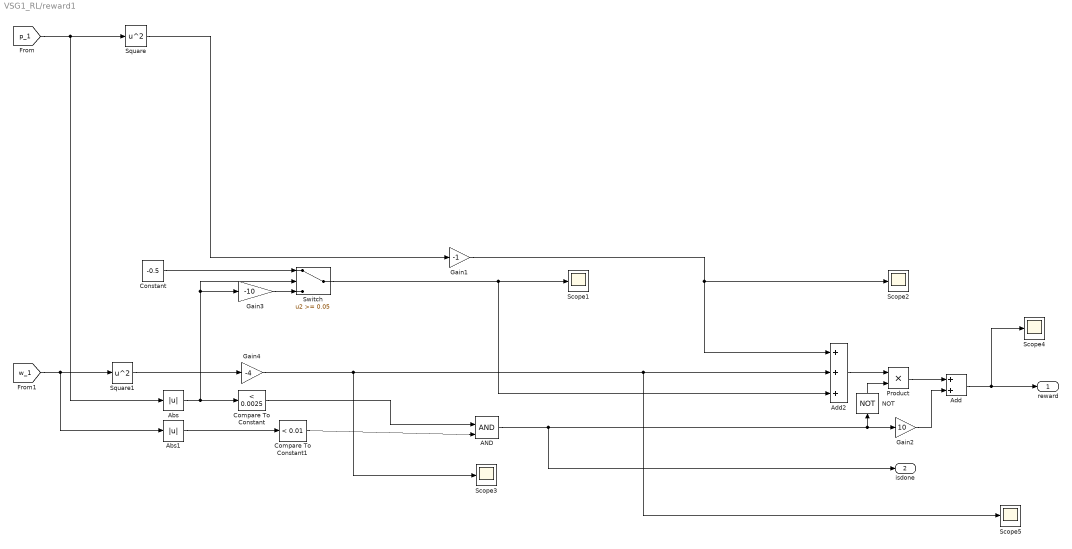
== system VSG1_RL/reward1 ==
  AND : Logic  IconShape=distinctive  AllPortsSameDT=off  OutDataTypeStr=boolean
  Abs : Abs  SaturateOnIntegerOverflow=off
  Abs1 : Abs  SaturateOnIntegerOverflow=off
  Add : Sum
  Add2 : Sum  Inputs=+++
  Compare To Constant : simulink/Logic and Bit Operations/Compare To Constant  relop=<  const=0.0025  OutDataTypeStr=boolean
  Compare To Constant1 : simulink/Logic and Bit Operations/Compare To Constant  relop=<  const=0.01  OutDataTypeStr=boolean
  Constant : Constant  Value=-0.5
  Gain1 : Gain  Gain=-1
  Gain2 : Gain  Gain=10
  Gain3 : Gain  Gain=-10
  Gain4 : Gain  Gain=-4
  NOT : Logic  Operator=NOT  IconShape=distinctive  AllPortsSameDT=off  OutDataTypeStr=boolean
  Product : Product
  Scope{1..5} (5 alike) : Scope
  Square : Math  Operator=square
  Square1 : Math  Operator=square
  Switch : Switch  Threshold=0.05  SaturateOnIntegerOverflow=off  InputSameDT=off
  reward : Outport
  isdone : Outport  Port=2
  wires:
  AND/1 -> NOT/1, Gain2/1, isdone/1
  Compare To Constant1/1 -> AND/2
  Square1/1 -> Gain4/1
  [w_1] -> Abs1/1, Square1/1
  Compare To Constant/1 -> AND/1
  Square/1 -> Gain1/1
  [p_1] -> Abs/1, Square/1
  Gain4/1 -> Scope3/1, Scope5/1, Add2/2
  Gain1/1 -> Scope2/1, Add2/1
  Abs/1 -> Gain3/1, Switch/2, Compare To Constant/1
  Abs1/1 -> Compare To Constant1/1
  Constant/1 -> Switch/1
  Gain3/1 -> Switch/3
  Switch/1 -> Add2/3, Scope1/1
  Add2/1 -> Product/1
  NOT/1 -> Product/2
  Product/1 -> Add/1
  Gain2/1 -> Add/2
  Add/1 -> Scope4/1, reward/1

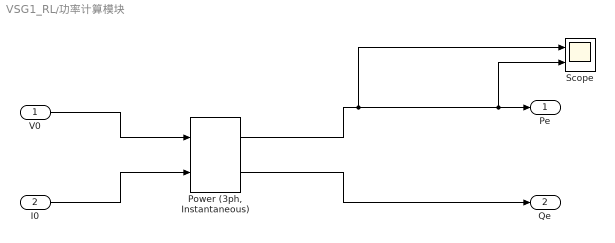
== system VSG1_RL/功率计算模块 ==
  V0 : Inport
  I0 : Inport  Port=2
  "Power (3ph, Instantaneous)" : spsPower3phInstantaneousLib/Power (3ph, Instantaneous)
  Scope : Scope  NumInputPorts=2
  Pe : Outport  VectorParamsAs1DForOutWhenUnconnected=off
  Qe : Outport  Port=2  VectorParamsAs1DForOutWhenUnconnected=off
  wires:
  V0/1 -> "Power (3ph, Instantaneous)"/1
  I0/1 -> "Power (3ph, Instantaneous)"/2
  "Power (3ph, Instantaneous)"/1 -> Scope/2, Pe/1, Scope/1
  "Power (3ph, Instantaneous)"/2 -> Qe/1

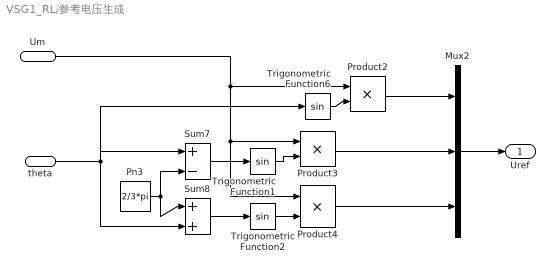
== system VSG1_RL/参考电压生成 ==
  Um : Inport
  theta : Inport  Port=2
  Mux2 : Mux  Inputs=3
  Pn3 : Constant  Value=2/3*pi
  Product2 : Product  RndMeth=Zero
  Product3 : Product  RndMeth=Zero
  Product4 : Product  RndMeth=Zero
  Sum7 : Sum  Inputs=|+-
  Sum8 : Sum  Inputs=|++
  Trigonometric Function1 : Trigonometry
  Trigonometric Function2 : Trigonometry
  Trigonometric Function6 : Trigonometry
  Uref : Outport  VectorParamsAs1DForOutWhenUnconnected=off
  wires:
  theta/1 -> Sum8/2, Sum7/1, Trigonometric Function6/1
  Product4/1 -> Mux2/3
  Product3/1 -> Mux2/2
  Product2/1 -> Mux2/1
  Mux2/1 -> Uref/1
  Um/1 -> Product2/1, Product3/1, Product4/1
  Trigonometric Function2/1 -> Product4/2
  Sum8/1 -> Trigonometric Function2/1
  Pn3/1 -> Sum8/1, Sum7/2
  Trigonometric Function1/1 -> Product3/2
  Sum7/1 -> Trigonometric Function1/1
  Trigonometric Function6/1 -> Product2/2

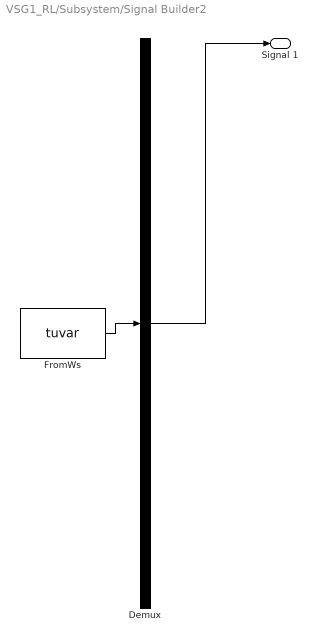
== system VSG1_RL/Subsystem/Signal Builder2 ==
  Demux : Demux  Tag=STV Demux  Outputs=1
      settings: DisplayOption=none
  FromWs : FromWorkspace  Tag=STV FromWs  VariableName=tuvar
      SigBuilderData=|
      | common.afterFinalStr = 'Extrapolate'
      | common.sampleTime = 0
      | dataSet.timeRange = [0 3]
      | dataSet.name = 'Group 1'
      | sbobj.Groups.Name = 'Group 1'
      | sbobj.Groups.Signals.Name = 'Signal 1'
      | sbobj.Groups.Signals.XData = [0 0.5 1.5 1.5 2.25 2.25 3]
      | sbobj.Groups.Signals.YData = [20000 20000 20000 0 0 20000 20000]
      | sbobj.Groups.TimeRange = [0 3]
  Signal 1 : Outport  Tag=STV Outport  VectorParamsAs1DForOutWhenUnconnected=off
  wires:
  FromWs/1 -> Demux/1
  Demux/1 -> Signal 1/1

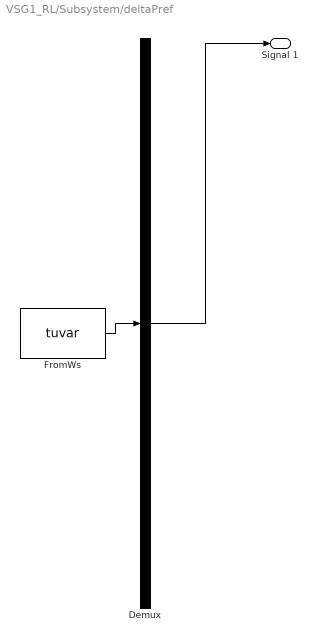
== system VSG1_RL/Subsystem/deltaPref ==
  Demux : Demux  Tag=STV Demux  Outputs=1
      settings: DisplayOption=none
  FromWs : FromWorkspace  Tag=STV FromWs  VariableName=tuvar
      SigBuilderData=|
      | common.afterFinalStr = 'Extrapolate'
      | common.sampleTime = 0
      | dataSet.timeRange = [0 3]
      | dataSet.name = 'Group 1'
      | sbobj.Groups.Name = 'Group 1'
      | sbobj.Groups.Signals.Name = 'Signal 1'
      | sbobj.Groups.Signals.XData = [0 0.5 1 1.5 3]
      | sbobj.Groups.Signals.YData = [20000 20000 20000 20000 20000]
      | sbobj.Groups.TimeRange = [0 3]
  Signal 1 : Outport  Tag=STV Outport  VectorParamsAs1DForOutWhenUnconnected=off
  wires:
  FromWs/1 -> Demux/1
  Demux/1 -> Signal 1/1

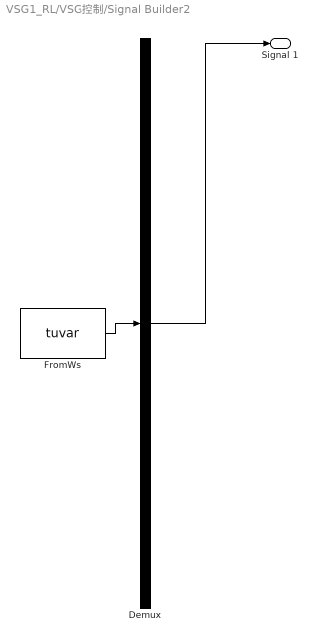
== system VSG1_RL/VSG控制/Signal Builder2 ==
  Demux : Demux  Tag=STV Demux  Outputs=1
      settings: DisplayOption=none
  FromWs : FromWorkspace  Tag=STV FromWs  VariableName=tuvar
      SigBuilderData=|
      | common.afterFinalStr = 'Extrapolate'
      | common.sampleTime = 0
      | dataSet.timeRange = [0 3]
      | dataSet.name = 'Group 1'
      | sbobj.Groups.Name = 'Group 1'
      | sbobj.Groups.Signals.Name = 'Signal 1'
      | sbobj.Groups.Signals.XData = [0 0.5 0.5 1.5 1.5 2.25 2.25 3]
      | sbobj.Groups.Signals.YData = [0 0 20000 20000 0 0 20000 20000]
      | sbobj.Groups.TimeRange = [0 3]
  Signal 1 : Outport  Tag=STV Outport  VectorParamsAs1DForOutWhenUnconnected=off
  wires:
  FromWs/1 -> Demux/1
  Demux/1 -> Signal 1/1
